simulink model "KUKA_KR6R900"  (R2024a)
settings: Solver=VariableStepAuto  StartTime=0.0  StopTime=30  RelTol=1e-3
undefined symbols (not defined in the file): X, Y, Z
libraries: sm_lib x37, fl_ps_legacy_lib x15, nesl_utility x12
(part 2 of 2)

== matlab function KUKA_KR6R900/xyzabc2mat/Euler to 3x3 ==
  data: angles input; R output; sequence input
function R = eulerToMatrix(angles, sequence)
% eulerToMatrix Converts Euler angles to a 3x3 rotation matrix with a specified sequence.
%
% INPUT:
% angles   - [3x1] vector of Euler angles [a1, a2, a3]
% sequence - Rotation sequence as a string, e.g., 'XYZ', 'ZYX'
% unit     - 'rad' or 'deg' (optional, default: 'rad')
%
% OUTPUT:
% R        - 3x3 Rotation matrix


% Precompute cos and sin
c = cos(angles);
s = sin(angles);

% Rotation matrix identities
R = eye(3);

%sequence_char = char(sequence);
sequence_char = sequence;
for i = 3:-1:1 % Reverse Loop Order
    axis = sequence_char(i);

    switch axis
        case 88
            Ri = [1, 0, 0; 0, c(i), -s(i); 0, s(i), c(i)];
        case 89
            Ri = [c(i), 0, s(i); 0, 1, 0; -s(i), 0, c(i)];
        case 90
            Ri = [c(i), -s(i), 0; s(i), c(i), 0; 0, 0, 1];
        otherwise
            error('Invalid axis');
    end
    R = Ri * R;
end

% Passive Rotation (Simulink style)
R = R';
end

== matlab function KUKA_KR6R900/Inverse kinematic/MATLAB Function1 ==
  data: T input; Q output; robot_param input
function Q = in_kinematics(T, robot_param)
% T - Extended 4x4 rotation and position matrix, or quaternion.
% The function provides 8 configuration options.
if size(T) == 4
    q = [[1; T(1:3, 4)] [0 0 0; T(1:3,1:3)]];
    [a] = ik_6Ropw(robot_param, q);
    Q = zeros(6, 8);
    Q = real(a) * 180 / pi;  % Convert radians to degrees
else
    error('Error: input argument must be a 4x4 matrix')
end

    function [theta] = ik_6Ropw(robot_param, EE)
    % Computes the inverse kinematics of serial manipulators
    % with an ortho-parallel basis and a spherical wrist.
    
    if nargin ~= 2
        error('Error: Not correct number of input arguments.')
    end
    
    if (size(EE, 1)) ~= 4
        error('Error: EE is not a homogeneous 4x4 matrix.')
    end
    
    % Proceed with inverse kinematics calculation...
    c4 = robot_param(7);
    C = [1 0 0 0; EE(2:4, 1) - EE(2:4, 4) * c4, EE(2:4, 2:4)];
    
    % Computing the first three angles
    theta123 = real(ik_3Ropw(robot_param, C(2:4, 1))); % Avoid rounding image part
    
    ind = find([isreal(theta123(:, 1)) isreal(theta123(:, 2)) isreal(theta123(:, 3)) isreal(theta123(:, 4))] == 1); % Indices where theta123 is real
    
    % Computing the second three angles
    c23 = cos(theta123(2, ind) + theta123(3, ind));
    s23 = sin(theta123(2, ind) + theta123(3, ind));
    
    r11 = EE(2, 2); r12 = EE(2, 3); r13 = EE(2, 4);
    r21 = EE(3, 2); r22 = EE(3, 3); r23 = EE(3, 4);
    r31 = EE(4, 2); r32 = EE(4, 3); r33 = EE(4, 4);
    
    M1 = ones(3, 4) * 1i; % Allocation
    
    if not(isempty(ind))
        M1(1, ind) = atan2(-r13 * sin(theta123(1, ind)) + r23 * cos(theta123(1, ind)), ...
                           r13 * cos(theta123(1, ind)) .* c23 + r23 * sin(theta123(1, ind)) .* c23 - r33 * s23);
        M1(2, ind) = atan2(sqrt(1 - (r13 * cos(theta123(1, ind)) .* s23 + r23 * sin(theta123(1, ind)) .* s23 + r33 * c23).^2), ...
                           r13 * cos(theta123(1, ind)) .* s23 + r23 * sin(theta123(1, ind)) .* s23 + r33 * c23);
        M1(3, ind) = atan2(r12 * cos(theta123(1, ind)) .* s23 + r22 * sin(theta123(1, ind)) .* s23 + r32 * c23, ...
                           -r11 * cos(theta123(1, ind)) .* s23 - r21 * sin(theta123(1, ind)) .* s23 - r31 * c23);
    end
    
    M2 = ones(3, 4) * 1i; % Allocation
    M2(1, :) = M1(1, :) + pi;
    M2(2, :) = -M1(2, :);
    M2(3, :) = M1(3, :) - pi;
    
    % Combine all possible solutions
    theta = [theta123(:, 1) theta123(:, 1) theta123(:, 2) theta123(:, 2) ...
             theta123(:, 3) theta123(:, 3) theta123(:, 4) theta123(:, 4);
             M1(:, 1) M2(:, 1) M1(:, 2) M2(:, 2) M1(:, 3) M2(:, 3) M1(:, 4) M2(:, 4)];
    
    %
    theta = real(theta);
    
    % Output cosmetics
    theta = theta + pi;  % Ensure that all angles are within [-pi, pi]
    theta = mod(real(theta), 2 * pi) + 1i * imag(theta);
    theta = theta - pi;
    end

    function theta = ik_3Ropw(robot_param, C)
    %theta = ik_3Ropw( robot_param, C )
    %   Computes the inverse kinematics of serial manipulators with an
    %   ortho-parallel basis.
    %
    %   robot_param ... [a1, a2, b1, c1, c2, c3, c4]
    %   C ... [cx0, cy0, cz0]
    %   theta is a matrix with all four possible solutions.
    
    a1 = robot_param(1);
    a2 = robot_param(2);
    b1 = robot_param(3);
    c1 = robot_param(4);
    c2 = robot_param(5);
    c3 = robot_param(6);
    
    cx0 = C(1);
    cy0 = C(2);
    cz0 = C(3);
    
    nx1 = sqrt(cx0^2 + cy0^2 - b1^2) - a1;
    s12 = nx1^2 + (cz0 - c1)^2; % s12 = s1^2
    s22 = (nx1 + 2 * a1)^2 + (cz0 - c1)^2; % s22 = s2^2
    k = sqrt(a2^2 + c3^2);

    theta = ones(3, 4) * 1i; % Allocation

    if isreal(nx1)
        if isreal(nx1 + a1)
            theta(1, 1) = atan2(cy0, cx0) - atan2(b1, nx1 + a1);
            theta(1, 2) = theta(1, 1);
            theta(1, 3) = atan2(cy0, cx0) + atan2(b1, nx1 + a1) - pi;
            theta(1, 4) = theta(1, 3);
        end % if

        theta(2, 1) = -acos((s12 + c2^2 - k^2) / (2 * sqrt(s12) * c2)) + atan2(nx1, cz0 - c1);
        theta(2, 2) = acos((s12 + c2^2 - k^2) / (2 * sqrt(s12) * c2)) + atan2(nx1, cz0 - c1);
        if isreal(nx1 + 2 * a1)
            theta(2, 3) = -acos((s22 + c2^2 - k^2) / (2 * sqrt(s22) * c2)) - atan2(nx1 + 2 * a1, cz0 - c1);
            theta(2, 4) = acos((s22 + c2^2 - k^2) / (2 * sqrt(s22) * c2)) - atan2(nx1 + 2 * a1, cz0 - c1);
        end % if

        theta(3, 1) = acos((s12 - c2^2 - k^2) / (2 * c2 * k)) - atan2(a2, c3);
        theta(3, 2) = -acos((s12 - c2^2 - k^2) / (2 * c2 * k)) - atan2(a2, c3);
        theta(3, 3) = acos((s22 - c2^2 - k^2) / (2 * c2 * k)) - atan2(a2, c3);
        theta(3, 4) = -acos((s22 - c2^2 - k^2) / (2 * c2 * k)) - atan2(a2, c3);

    end % if
end
end

== matlab function KUKA_KR6R900/xyzabc2mat/MATLAB Function ==
  data: orientation input; matrix output; XYZ input
function matrix = fcn(orientation, XYZ)
q=[XYZ(1),XYZ(2),XYZ(3),  1]';
orientation=[orientation; 0 0 0];
matrix=[orientation q];
